simulink model "VehiclePlant"  (R2024b)
settings: Solver=VariableStepAuto  StartTime=0.0  StopTime=300  RelTol=1e-3
undefined symbols (not defined in the file): A_f, C_D, Crr, d_0, d_max, d_min, g, m, rho, t_headway, v_0
libraries: simulink x6, simulink_extras x1, mpclib x1
settings Model: Creator=User  LastModifiedBy=User

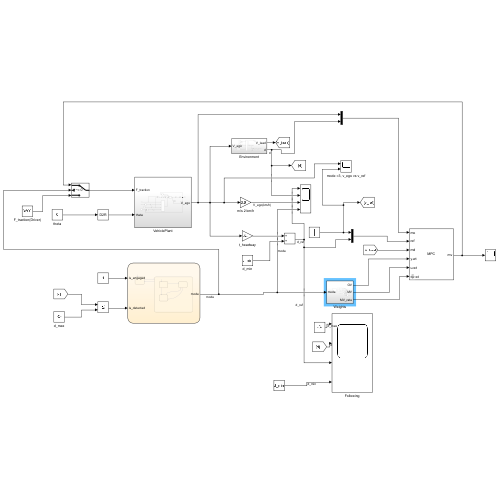
[thumbnail: Simulink's stored preview of the top-level diagram]
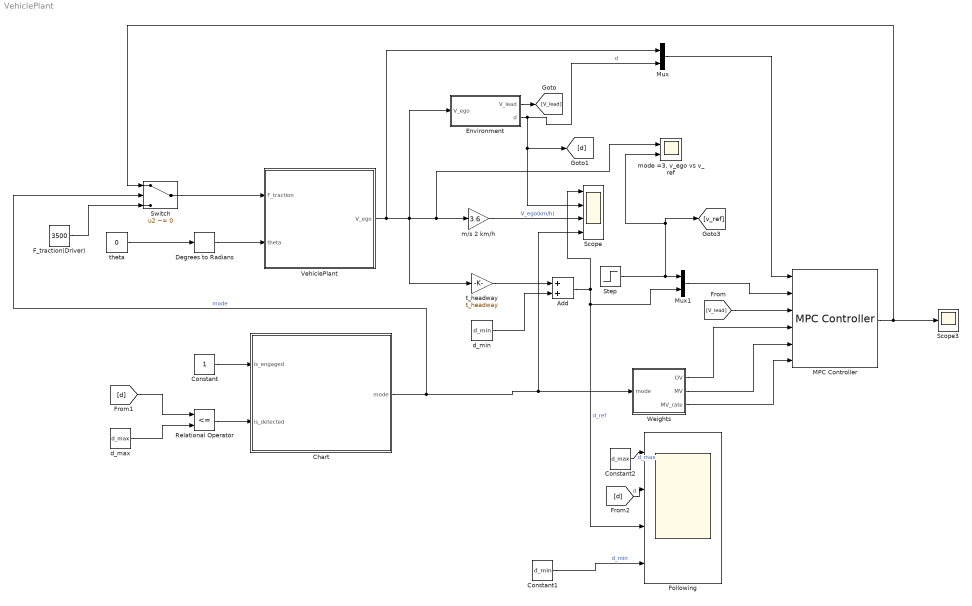
== system VehiclePlant ==
  Add : Sum
  Chart : Stateflow chart  TreatAsAtomicUnit=on
  Constant : Constant
  Constant1 : Constant  Value=d_min
  Constant2 : Constant  Value=d_max
  Degrees to Radians : simulink_extras/Transformations/Degrees to Radians
  Environment : Subsystem
  F_traction(Driver) : Constant  Value=3500
  Following : Scope  NumInputPorts=4
  MPC Controller : mpclib/MPC Controller  SCDEnableBlockLinearizationSpecification=on  mpcobj=mpcobj  is_multiple=0  enable_value=0  return_u0=off  updateMPCinCallerWorkspace=on  md_inport=on  mv_inport=off  uref_inport=off  return_cost=off  return_mvseq=off  return_qpstatus=off  return_xseq=off  return_state=off  return_ovseq=off  state_inport=off  umin_inport=off  umax_inport=off  ymin_inport=off  ymax_inport=off  cc_inport=off  ywt_inport=on  uwt_inport=on  duwt_inport=on  rhoeps_inport=off  pm_inport=off  MaximumP=10  HorizonChoice=FixedHorizon  n_ts=0.1  n_p=50  n_mv=1  n_md=1  n_ud=0  n_mo=2  n_uo=0  BlockDataType=double  SampleTimeInherited=off  switch_inport=off
  Mux : Mux  Inputs=2
  Mux1 : Mux  Inputs=2
  Relational Operator : RelationalOperator  Operator=<=  OutDataTypeStr=boolean  RndMeth=Simplest  InputSameDT=off
  Scope : Scope  NumInputPorts=4
  Scope3 : Scope
  Step : Step  Time=50  After=80/3.6  SampleTime=0
  Switch : Switch  Criteria=u2 ~= 0  SaturateOnIntegerOverflow=off  InputSameDT=off
  VehiclePlant : Subsystem
  Weights : Subsystem
  d_max : Constant  Value=d_max
  d_min : Constant  Value=d_min
  m/s 2 km/h : Gain  Gain=3.6
  "mode =3, v_ego vs v_ref" : Scope  NumInputPorts=2
  t_headway : Gain  Gain=t_headway
  theta : Constant  Value=0
  wires:
  theta/1 -> Degrees to Radians/1
  VehiclePlant/1(V_ego) -> Mux/1, t_headway/1, Environment/1(V_ego), "mode =3, v_ego vs v_ref"/1, m/s 2 km/h/1
  Degrees to Radians/1 -> VehiclePlant/2(theta)
  Environment/2(d) -> [d], Scope/2, Mux/2  "d"
  Mux1/1 -> MPC Controller/2
  Add/1 -> Scope/1, Mux1/2, Following/3  "d_ref"
  d_min/1 -> Add/2
  t_headway/1 -> Add/1
  Environment/1(V_lead) -> [V_lead]
  [V_lead] -> MPC Controller/3
  MPC Controller/1 -> Scope3/1, Switch/1
  Mux/1 -> MPC Controller/1
  Weights/1(OV) -> MPC Controller/4
  Step/1 -> "mode =3, v_ego vs v_ref"/2, [v_ref], Mux1/1
  Weights/2(MV) -> MPC Controller/5
  Weights/3(MV_rate) -> MPC Controller/6
  Chart/1(mode) -> Switch/2, Weights/1(mode), Scope/4  "mode"
  Constant/1 -> Chart/1(is_engaged)
  d_max/1 -> Relational Operator/2
  [d] -> Relational Operator/1
  m/s 2 km/h/1 -> Scope/3  "V_ego(km/h)"
  Relational Operator/1 -> Chart/2(is_detected)
  Switch/1 -> VehiclePlant/1(F_traction)
  F_traction(Driver)/1 -> Switch/3
  [d] -> Following/2  "d"
  Constant2/1 -> Following/1  "d_max"
  Constant1/1 -> Following/4  "d_min"

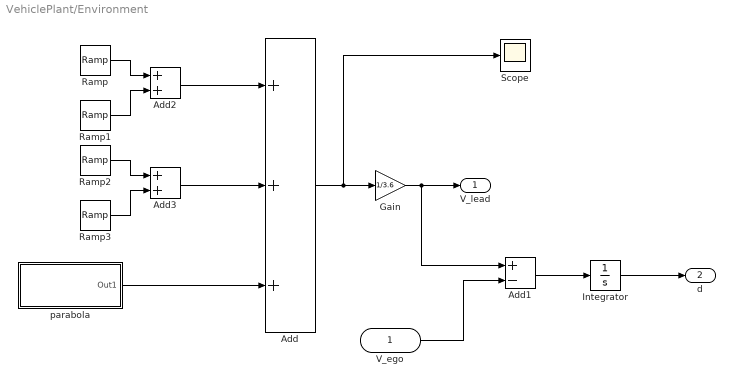
== system VehiclePlant/Environment ==
  V_ego : Inport
  Add : Sum  Inputs=+++
  Add1 : Sum  Inputs=+-
  Add2 : Sum
  Add3 : Sum
  Gain : Gain  Gain=1/3.6
  Integrator : Integrator  InitialCondition=d_0
  Ramp : simulink/Sources/Ramp  slope=2  start=0  InitialOutput=0
  Ramp1 : simulink/Sources/Ramp  slope=-2  start=30  InitialOutput=0
  Ramp2 : simulink/Sources/Ramp  slope=1  start=90  InitialOutput=0
  Ramp3 : simulink/Sources/Ramp  slope=-1  start=150  InitialOutput=0
  Scope : Scope
  parabola : Subsystem
  V_lead : Outport
  d : Outport  Port=2
  wires:
  Add/1 -> Scope/1, Gain/1
  Gain/1 -> Add1/1, V_lead/1
  V_ego/1 -> Add1/2
  Add1/1 -> Integrator/1
  Integrator/1 -> d/1
  parabola/1(Out1) -> Add/3
  Ramp1/1 -> Add2/2
  Ramp/1 -> Add2/1
  Ramp2/1 -> Add3/1
  Ramp3/1 -> Add3/2
  Add3/1 -> Add/2
  Add2/1 -> Add/1

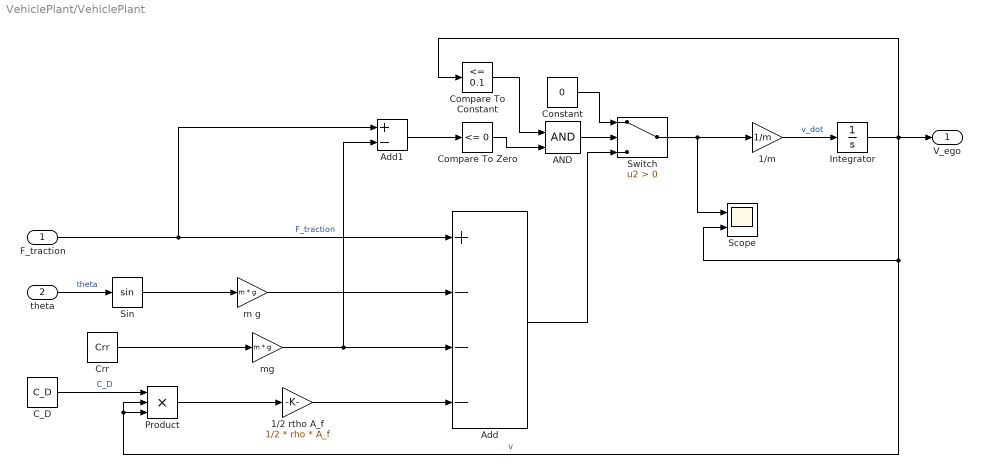
== system VehiclePlant/VehiclePlant ==
  F_traction : Inport
  theta : Inport  Port=2
  1/2 rtho A_f : Gain  Gain=1/2 * rho * A_f
  1/m : Gain  Gain=1/m
  AND : Logic  IconShape=distinctive  AllPortsSameDT=off  OutDataTypeStr=boolean
  Add : Sum  Inputs=+---
  Add1 : Sum  Inputs=+-
  C_D : Constant  Value=C_D
  Compare To Constant : simulink/Logic and Bit Operations/Compare To Constant  relop=<=  const=0.1  OutDataTypeStr=boolean
  Compare To Zero : simulink/Logic and Bit Operations/Compare To Zero  relop=<=  OutDataTypeStr=boolean
  Constant : Constant  Value=0
  Crr : Constant  Value=Crr
  Integrator : Integrator  InitialCondition=v_0
  Product : Product  Inputs=3
  Scope : Scope  NumInputPorts=2
  Sin : Trigonometry
  Switch : Switch  Criteria=u2 > Threshold  SaturateOnIntegerOverflow=off  InputSameDT=off
  m g : Gain  Gain=m * g
  mg : Gain  Gain=m * g
  V_ego : Outport
  wires:
  1/m/1 -> Integrator/1  "v_dot"
  Integrator/1 -> Compare To Constant/1, V_ego/1, Scope/2, Product/2, Product/3  "v"
  F_traction/1 -> Add1/1, Add/1  "F_traction"
  Product/1 -> 1/2 rtho A_f/1
  1/2 rtho A_f/1 -> Add/4
  theta/1 -> Sin/1  "theta"
  Sin/1 -> m g/1
  m g/1 -> Add/2
  C_D/1 -> Product/1  "C_D"
  mg/1 -> Add1/2, Add/3
  Crr/1 -> mg/1
  Add1/1 -> Compare To Zero/1
  Switch/1 -> Scope/1, 1/m/1
  Add/1 -> Switch/3
  Constant/1 -> Switch/1
  Compare To Constant/1 -> AND/1
  Compare To Zero/1 -> AND/2
  AND/1 -> Switch/2

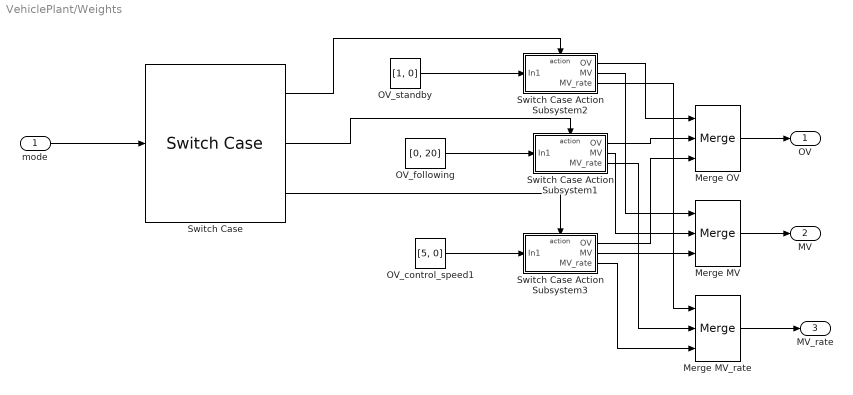
== system VehiclePlant/Weights ==
  mode : Inport
  Merge MV : Merge  Inputs=3
  Merge MV_rate : Merge  Inputs=3
  Merge OV : Merge  Inputs=3
  OV_control_speed1 : Constant  Value=[5, 0]
  OV_following : Constant  Value=[0, 20]
  OV_standby : Constant  Value=[1, 0]
  Switch Case : SwitchCase  CaseConditions={1, 2, 3}  ShowDefaultCase=off
  Switch Case Action Subsystem1 : Subsystem  TreatAsAtomicUnit=on
  Switch Case Action Subsystem2 : Subsystem  TreatAsAtomicUnit=on
  Switch Case Action Subsystem3 : Subsystem  TreatAsAtomicUnit=on
  OV : Outport
  MV : Outport  Port=2
  MV_rate : Outport  Port=3
  wires:
  Switch Case/1 -> Switch Case Action Subsystem2/Action
  Switch Case/3 -> Switch Case Action Subsystem3/Action
  OV_standby/1 -> Switch Case Action Subsystem2/1(In1)
  OV_following/1 -> Switch Case Action Subsystem1/1(In1)
  OV_control_speed1/1 -> Switch Case Action Subsystem3/1(In1)
  mode/1 -> Switch Case/1
  Merge OV/1 -> OV/1
  Merge MV_rate/1 -> MV_rate/1
  Merge MV/1 -> MV/1
  Switch Case Action Subsystem3/1(OV) -> Merge OV/3
  Switch Case Action Subsystem1/1(OV) -> Merge OV/2
  Switch Case Action Subsystem2/1(OV) -> Merge OV/1
  Switch Case Action Subsystem2/2(MV) -> Merge MV/1
  Switch Case Action Subsystem1/2(MV) -> Merge MV/2
  Switch Case Action Subsystem3/2(MV) -> Merge MV/3
  Switch Case Action Subsystem2/3(MV_rate) -> Merge MV_rate/1
  Switch Case Action Subsystem1/3(MV_rate) -> Merge MV_rate/2
  Switch Case Action Subsystem3/3(MV_rate) -> Merge MV_rate/3
  Switch Case/2 -> Switch Case Action Subsystem1/Action

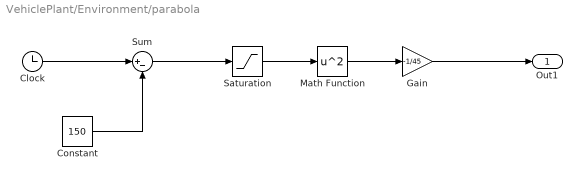
== system VehiclePlant/Environment/parabola ==
  Clock : Clock
  Constant : Constant  Value=150
  Gain : Gain  Gain=-1/45
  Math Function : Math  Operator=square
  Saturation : Saturate  UpperLimit=60  LowerLimit=0
  Sum : Sum  Inputs=|+-
  Out1 : Outport
  wires:
  Clock/1 -> Sum/1
  Constant/1 -> Sum/2
  Sum/1 -> Saturation/1
  Saturation/1 -> Math Function/1
  Math Function/1 -> Gain/1
  Gain/1 -> Out1/1

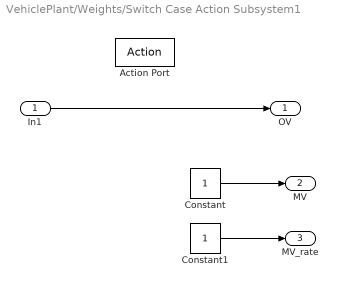
== system VehiclePlant/Weights/Switch Case Action Subsystem1 ==
  In1 : Inport
  Action Port : ActionPort  ActionPortLabel=case [ 2 ]:
  Constant : Constant
  Constant1 : Constant
  OV : Outport
  MV : Outport  Port=2
  MV_rate : Outport  Port=3
  wires:
  In1/1 -> OV/1
  Constant/1 -> MV/1
  Constant1/1 -> MV_rate/1

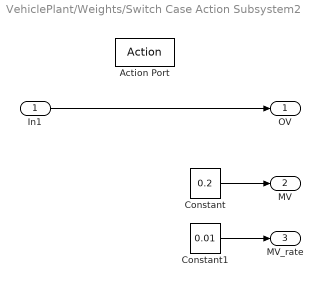
== system VehiclePlant/Weights/Switch Case Action Subsystem2 ==
  In1 : Inport
  Action Port : ActionPort  ActionPortLabel=case [ 1 ]:
  Constant : Constant  Value=0.2
  Constant1 : Constant  Value=0.01
  OV : Outport
  MV : Outport  Port=2
  MV_rate : Outport  Port=3
  wires:
  In1/1 -> OV/1
  Constant/1 -> MV/1
  Constant1/1 -> MV_rate/1

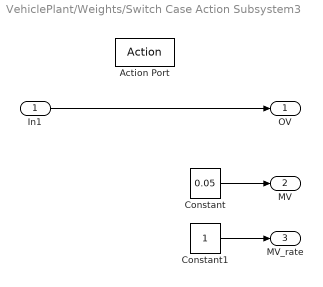
== system VehiclePlant/Weights/Switch Case Action Subsystem3 ==
  In1 : Inport
  Action Port : ActionPort  ActionPortLabel=case [ 3 ]:
  Constant : Constant  Value=0.05
  Constant1 : Constant
  OV : Outport
  MV : Outport  Port=2
  MV_rate : Outport  Port=3
  wires:
  In1/1 -> OV/1
  Constant/1 -> MV/1
  Constant1/1 -> MV_rate/1

== stateflow chart VehiclePlant/Chart ==
  state ACC_OFF
    entry: mode = 0;
  state ACC_ON
    state Standby
      entry: mode = 1;
    state Following
      entry: mode = 2;
    state Speed_Control
      entry: mode = 3;
    (default) -> Standby
    Standby -> Following [order 2] : [is_detected == 1]
    Standby -> Speed_Control [order 1] : [is_detected == 0]
    Speed_Control -> Following : [is_detected == 1]
    Following -> Speed_Control : [is_detected == 0]
  (default) -> ACC_OFF
  ACC_OFF -> ACC_ON : [is_engaged == 1]
  ACC_ON -> ACC_OFF : [is_engaged == 0]
  data: is_engaged input; is_detected input; mode output
